simulink model "AB_Final_of_MPC_Bandwidth_Result_UnbalancedNew"  (R2022b)
settings: Solver=FixedStepDiscrete  StartTime=0.0  StopTime=Inf  FixedStep=100e-6  RelTol=1e-3  EnableMultiTasking=on
undefined symbols (not defined in the file): C28x, CPU1, CPU2, CurrentBypassValue, DiscIntNeverNeededParam, Down, GPTRIP1SEL, TZ1, Up
libraries: c2802xlib x20, simulink x17, dspstat3 x13, eeGeneralControl x10, c2837xDlib x5, c280xlib x5, PID_Lib x4, c2000lib x1, spsAlphaBetaZerotoabcLib x1
(part 8 of 10)

== system AB_Final_of_MPC_Bandwidth_Result_UnbalancedNew/Subsystem1/GridCurrentSecondPrediction/CostFunctionofVoltageVectors/CostFunctionVoltage4 ==
  MPCC_f32DGridCurrent_K_1 : Inport
  MPCC_f32QGridCurrent_K_1 : Inport  Port=2
  MPCC_f32DGridVoltage : Inport  Port=3
  MPCC_f32QGridVoltage : Inport  Port=4
  MPCC_f32Predictionterm_A : Inport  Port=5
  MPCC_f32Predictionterm_B : Inport  Port=6
  MPCC_f32Predictionterm_C : Inport  Port=7
  MPCC_f32DGridCurrentReference : Inport  Port=8
  MPCC_f32QGridCurrentReference : Inport  Port=9
  MPCC_f32DVoltageVector4 : Inport  Port=10
  MPCC_f32QVoltageVector4 : Inport  Port=11
  MPCC_f32DGridCurrent : Inport  Port=12
  MPCC_f32QGridCurrent : Inport  Port=13
  MPCC_f32DGridCurrent1 : Inport  Port=14
  MPCC_f32QGridCurrent1 : Inport  Port=15
  CostFunctionVoltage4 : Subsystem
  DGridCurrentSecondPrediction_Voltage4 : Subsystem
  QGridCurrentSecondPrediction_Voltage4 : Subsystem
  MPCC_f32CostFunction_Voltage4 : Outport
  wires:
  [MPCC_f32Predictionterm_B] -> QGridCurrentSecondPrediction_Voltage4/2(MPCC_f32Predictionterm_B)
  [MPCC_f32QGridCurrent_K_1] -> DGridCurrentSecondPrediction_Voltage4/5(MPCC_f32QGridCurrent_K_1)
  [MPCC_f32Predictionterm_A] -> QGridCurrentSecondPrediction_Voltage4/1(MPCC_f32Predictionterm_A)
  [MPCC_f32QGridCurrent_K_1] -> QGridCurrentSecondPrediction_Voltage4/5(MPCC_f32QGridCurrent_K_1)
  [MPCC_f32Predictionterm_B] -> DGridCurrentSecondPrediction_Voltage4/2(MPCC_f32Predictionterm_B)
  [MPCC_f32DGridCurrent_K_1] -> QGridCurrentSecondPrediction_Voltage4/4(MPCC_f32DGridCurrent_K_1)
  [MPCC_f32Predictionterm_C] -> QGridCurrentSecondPrediction_Voltage4/3(MPCC_f32Predictionterm_C)
  [MPCC_f32Predictionterm_A] -> DGridCurrentSecondPrediction_Voltage4/1(MPCC_f32Predictionterm_A)
  DGridCurrentSecondPrediction_Voltage4/1(MPCC_f32DGridCurrent_K_2_Voltage4) -> [MPCC_f32DGridCurrent_K_2_Voltage4]
  [MPCC_f32Predictionterm_C] -> DGridCurrentSecondPrediction_Voltage4/3(MPCC_f32Predictionterm_C)
  [MPCC_f32QGridVoltage] -> QGridCurrentSecondPrediction_Voltage4/6(MPCC_f32QGridVoltage)
  [MPCC_f32DGridVoltage] -> DGridCurrentSecondPrediction_Voltage4/6(MPCC_f32DGridVoltage)
  [MPCC_f32DGridCurrent_K_1] -> DGridCurrentSecondPrediction_Voltage4/4(MPCC_f32DGridCurrent_K_1)
  MPCC_f32QGridVoltage/1 -> [MPCC_f32QGridVoltage]
  MPCC_f32DGridCurrent_K_1/1 -> [MPCC_f32DGridCurrent_K_1]
  MPCC_f32Predictionterm_A/1 -> [MPCC_f32Predictionterm_A]
  MPCC_f32DGridVoltage/1 -> [MPCC_f32DGridVoltage]
  MPCC_f32Predictionterm_C/1 -> [MPCC_f32Predictionterm_C]
  MPCC_f32QGridCurrent_K_1/1 -> [MPCC_f32QGridCurrent_K_1]
  MPCC_f32Predictionterm_B/1 -> [MPCC_f32Predictionterm_B]
  MPCC_f32DGridCurrentReference/1 -> [MPCC_f32DGridCurrentReference]
  MPCC_f32QGridCurrentReference/1 -> [MPCC_f32QGridCurrentReference]
  QGridCurrentSecondPrediction_Voltage4/1(MPCC_f32QGridCurrent_K_2_Voltage4) -> [MPCC_f32QGridCurrent_K_2_Voltage4]
  CostFunctionVoltage4/1(MPCC_f32CostFunction_Voltage4) -> MPCC_f32CostFunction_Voltage4/1
  [MPCC_f32DGridCurrentReference] -> CostFunctionVoltage4/1(MPCC_f32DGridCurrentReference)
  [MPCC_f32QGridCurrentReference] -> CostFunctionVoltage4/2(MPCC_f32QGridCurrentReference)
  [MPCC_f32DGridCurrent_K_2_Voltage4] -> CostFunctionVoltage4/3(MPCC_f32DGridCurrent_K_2_Voltage4)
  [MPCC_f32QGridCurrent_K_2_Voltage4] -> CostFunctionVoltage4/4(MPCC_f32QGridCurrent_K_2_Voltage4)
  [MPCC_f32DGridCurrent] -> CostFunctionVoltage4/5(MPCC_f32DGridCurrent)
  [MPCC_f32QGridCurrent] -> CostFunctionVoltage4/6(MPCC_f32QGridCurrent)
  [MPCC_f32DVoltageVector4] -> DGridCurrentSecondPrediction_Voltage4/7(MPCC_f32DVoltageVector4)
  [MPCC_f32QVoltageVector4] -> QGridCurrentSecondPrediction_Voltage4/7(MPCC_f32QVoltageVector4)
  MPCC_f32DVoltageVector4/1 -> [MPCC_f32DVoltageVector4]
  MPCC_f32QVoltageVector4/1 -> [MPCC_f32QVoltageVector4]
  MPCC_f32QGridCurrent/1 -> [MPCC_f32QGridCurrent]
  MPCC_f32DGridCurrent/1 -> [MPCC_f32DGridCurrent]
  MPCC_f32DGridCurrent1/1 -> CostFunctionVoltage4/7(MPCC_f32DGridCurrent1)
  MPCC_f32QGridCurrent1/1 -> CostFunctionVoltage4/8(MPCC_f32QGridCurrent1)

== system AB_Final_of_MPC_Bandwidth_Result_UnbalancedNew/Subsystem1/GridCurrentSecondPrediction/CostFunctionofVoltageVectors/CostFunctionVoltage5 ==
  MPCC_f32DGridCurrent_K_1 : Inport
  MPCC_f32QGridCurrent_K_1 : Inport  Port=2
  MPCC_f32DGridVoltage : Inport  Port=3
  MPCC_f32QGridVoltage : Inport  Port=4
  MPCC_f32Predictionterm_A : Inport  Port=5
  MPCC_f32Predictionterm_B : Inport  Port=6
  MPCC_f32Predictionterm_C : Inport  Port=7
  MPCC_f32DGridCurrentReference : Inport  Port=8
  MPCC_f32QGridCurrentReference : Inport  Port=9
  MPCC_f32DVoltageVector5 : Inport  Port=10
  MPCC_f32QVoltageVector5 : Inport  Port=11
  MPCC_f32DGridCurrent : Inport  Port=12
  MPCC_f32QGridCurrent : Inport  Port=13
  MPCC_f32DGridCurrent1 : Inport  Port=14
  MPCC_f32QGridCurrent1 : Inport  Port=15
  CostFunctionVoltage5 : Subsystem
  DGridCurrentSecondPrediction_Voltage5 : Subsystem
  QGridCurrentSecondPrediction_Voltage5 : Subsystem
  MPCC_f32CostFunction_Voltage5 : Outport
  wires:
  [MPCC_f32Predictionterm_B] -> QGridCurrentSecondPrediction_Voltage5/2(MPCC_f32Predictionterm_B)
  [MPCC_f32QGridCurrent_K_1] -> DGridCurrentSecondPrediction_Voltage5/5(MPCC_f32QGridCurrent_K_1)
  [MPCC_f32Predictionterm_A] -> QGridCurrentSecondPrediction_Voltage5/1(MPCC_f32Predictionterm_A)
  [MPCC_f32QGridCurrent_K_1] -> QGridCurrentSecondPrediction_Voltage5/5(MPCC_f32QGridCurrent_K_1)
  [MPCC_f32Predictionterm_B] -> DGridCurrentSecondPrediction_Voltage5/2(MPCC_f32Predictionterm_B)
  [MPCC_f32DGridCurrent_K_1] -> QGridCurrentSecondPrediction_Voltage5/4(MPCC_f32DGridCurrent_K_1)
  [MPCC_f32Predictionterm_C] -> QGridCurrentSecondPrediction_Voltage5/3(MPCC_f32Predictionterm_C)
  [MPCC_f32Predictionterm_A] -> DGridCurrentSecondPrediction_Voltage5/1(MPCC_f32Predictionterm_A)
  DGridCurrentSecondPrediction_Voltage5/1(MPCC_f32DGridCurrent_K_2_Voltage5) -> [MPCC_f32DGridCurrent_K_2_Voltage5]
  [MPCC_f32Predictionterm_C] -> DGridCurrentSecondPrediction_Voltage5/3(MPCC_f32Predictionterm_C)
  [MPCC_f32QGridVoltage] -> QGridCurrentSecondPrediction_Voltage5/6(MPCC_f32QGridVoltage)
  [MPCC_f32DGridVoltage] -> DGridCurrentSecondPrediction_Voltage5/6(MPCC_f32DGridVoltage)
  [MPCC_f32DGridCurrent_K_1] -> DGridCurrentSecondPrediction_Voltage5/4(MPCC_f32DGridCurrent_K_1)
  MPCC_f32QGridVoltage/1 -> [MPCC_f32QGridVoltage]
  MPCC_f32DGridCurrent_K_1/1 -> [MPCC_f32DGridCurrent_K_1]
  MPCC_f32Predictionterm_A/1 -> [MPCC_f32Predictionterm_A]
  MPCC_f32DGridVoltage/1 -> [MPCC_f32DGridVoltage]
  MPCC_f32Predictionterm_C/1 -> [MPCC_f32Predictionterm_C]
  MPCC_f32QGridCurrent_K_1/1 -> [MPCC_f32QGridCurrent_K_1]
  MPCC_f32Predictionterm_B/1 -> [MPCC_f32Predictionterm_B]
  MPCC_f32DGridCurrentReference/1 -> [MPCC_f32DGridCurrentReference]
  MPCC_f32QGridCurrentReference/1 -> [MPCC_f32QGridCurrentReference]
  QGridCurrentSecondPrediction_Voltage5/1(MPCC_f32QGridCurrent_K_2_Voltage5) -> [MPCC_f32QGridCurrent_K_2_Voltage5]
  CostFunctionVoltage5/1(MPCC_f32CostFunction_Voltage5) -> MPCC_f32CostFunction_Voltage5/1
  [MPCC_f32DGridCurrentReference] -> CostFunctionVoltage5/1(MPCC_f32DGridCurrentReference)
  [MPCC_f32QGridCurrentReference] -> CostFunctionVoltage5/2(MPCC_f32QGridCurrentReference)
  [MPCC_f32DGridCurrent_K_2_Voltage5] -> CostFunctionVoltage5/3(MPCC_f32DGridCurrent_K_2_Voltage5)
  [MPCC_f32QGridCurrent_K_2_Voltage5] -> CostFunctionVoltage5/4(MPCC_f32QGridCurrent_K_2_Voltage5)
  [MPCC_f32DGridCurrent] -> CostFunctionVoltage5/5(MPCC_f32DGridCurrent)
  [MPCC_f32QGridCurrent] -> CostFunctionVoltage5/6(MPCC_f32QGridCurrent)
  [MPCC_f32DVoltageVector5] -> DGridCurrentSecondPrediction_Voltage5/7(MPCC_f32DVoltageVector5)
  [MPCC_f32QVoltageVector5] -> QGridCurrentSecondPrediction_Voltage5/7(MPCC_f32QVoltageVector5)
  MPCC_f32DVoltageVector5/1 -> [MPCC_f32DVoltageVector5]
  MPCC_f32QVoltageVector5/1 -> [MPCC_f32QVoltageVector5]
  MPCC_f32QGridCurrent/1 -> [MPCC_f32QGridCurrent]
  MPCC_f32DGridCurrent/1 -> [MPCC_f32DGridCurrent]
  MPCC_f32DGridCurrent1/1 -> CostFunctionVoltage5/7(MPCC_f32DGridCurrent1)
  MPCC_f32QGridCurrent1/1 -> CostFunctionVoltage5/8(MPCC_f32QGridCurrent1)

== system AB_Final_of_MPC_Bandwidth_Result_UnbalancedNew/Subsystem1/GridCurrentSecondPrediction/CostFunctionofVoltageVectors/CostFunctionVoltage6 ==
  MPCC_f32DGridCurrent_K_1 : Inport
  MPCC_f32QGridCurrent_K_1 : Inport  Port=2
  MPCC_f32DGridVoltage : Inport  Port=3
  MPCC_f32QGridVoltage : Inport  Port=4
  MPCC_f32Predictionterm_A : Inport  Port=5
  MPCC_f32Predictionterm_B : Inport  Port=6
  MPCC_f32Predictionterm_C : Inport  Port=7
  MPCC_f32DGridCurrentReference : Inport  Port=8
  MPCC_f32QGridCurrentReference : Inport  Port=9
  MPCC_f32DVoltageVector6 : Inport  Port=10
  MPCC_f32QVoltageVector6 : Inport  Port=11
  MPCC_f32DGridCurrent : Inport  Port=12
  MPCC_f32QGridCurrent : Inport  Port=13
  MPCC_f32DGridCurrent1 : Inport  Port=14
  MPCC_f32QGridCurrent1 : Inport  Port=15
  CostFunctionVoltage6 : Subsystem
  DGridCurrentSecondPrediction_Voltage6 : Subsystem
  QGridCurrentSecondPrediction_Voltage6 : Subsystem
  MPCC_f32CostFunction_Voltage6 : Outport
  wires:
  [MPCC_f32Predictionterm_B] -> QGridCurrentSecondPrediction_Voltage6/2(MPCC_f32Predictionterm_B)
  [MPCC_f32QGridCurrent_K_1] -> DGridCurrentSecondPrediction_Voltage6/5(MPCC_f32QGridCurrent_K_1)
  [MPCC_f32Predictionterm_A] -> QGridCurrentSecondPrediction_Voltage6/1(MPCC_f32Predictionterm_A)
  [MPCC_f32QGridCurrent_K_1] -> QGridCurrentSecondPrediction_Voltage6/5(MPCC_f32QGridCurrent_K_1)
  [MPCC_f32Predictionterm_B] -> DGridCurrentSecondPrediction_Voltage6/2(MPCC_f32Predictionterm_B)
  [MPCC_f32DGridCurrent_K_1] -> QGridCurrentSecondPrediction_Voltage6/4(MPCC_f32DGridCurrent_K_1)
  [MPCC_f32Predictionterm_C] -> QGridCurrentSecondPrediction_Voltage6/3(MPCC_f32Predictionterm_C)
  [MPCC_f32Predictionterm_A] -> DGridCurrentSecondPrediction_Voltage6/1(MPCC_f32Predictionterm_A)
  DGridCurrentSecondPrediction_Voltage6/1(MPCC_f32DGridCurrent_K_2_Voltage6) -> [MPCC_f32DGridCurrent_K_2_Voltage6]
  [MPCC_f32Predictionterm_C] -> DGridCurrentSecondPrediction_Voltage6/3(MPCC_f32Predictionterm_C)
  [MPCC_f32QGridVoltage] -> QGridCurrentSecondPrediction_Voltage6/6(MPCC_f32QGridVoltage)
  [MPCC_f32DGridVoltage] -> DGridCurrentSecondPrediction_Voltage6/6(MPCC_f32DGridVoltage)
  [MPCC_f32DGridCurrent_K_1] -> DGridCurrentSecondPrediction_Voltage6/4(MPCC_f32DGridCurrent_K_1)
  MPCC_f32QGridVoltage/1 -> [MPCC_f32QGridVoltage]
  MPCC_f32DGridCurrent_K_1/1 -> [MPCC_f32DGridCurrent_K_1]
  MPCC_f32Predictionterm_A/1 -> [MPCC_f32Predictionterm_A]
  MPCC_f32DGridVoltage/1 -> [MPCC_f32DGridVoltage]
  MPCC_f32Predictionterm_C/1 -> [MPCC_f32Predictionterm_C]
  MPCC_f32QGridCurrent_K_1/1 -> [MPCC_f32QGridCurrent_K_1]
  MPCC_f32Predictionterm_B/1 -> [MPCC_f32Predictionterm_B]
  MPCC_f32DGridCurrentReference/1 -> [MPCC_f32DGridCurrentReference]
  MPCC_f32QGridCurrentReference/1 -> [MPCC_f32QGridCurrentReference]
  QGridCurrentSecondPrediction_Voltage6/1(MPCC_f32QGridCurrent_K_2_Voltage6) -> [MPCC_f32QGridCurrent_K_2_Voltage6]
  CostFunctionVoltage6/1(MPCC_f32CostFunction_Voltage6) -> MPCC_f32CostFunction_Voltage6/1
  [MPCC_f32DGridCurrentReference] -> CostFunctionVoltage6/1(MPCC_f32DGridCurrentReference)
  [MPCC_f32QGridCurrentReference] -> CostFunctionVoltage6/2(MPCC_f32QGridCurrentReference)
  [MPCC_f32DGridCurrent_K_2_Voltage6] -> CostFunctionVoltage6/3(MPCC_f32DGridCurrent_K_2_Voltage6)
  [MPCC_f32QGridCurrent_K_2_Voltage6] -> CostFunctionVoltage6/4(MPCC_f32QGridCurrent_K_2_Voltage6)
  [MPCC_f32DGridCurrent] -> CostFunctionVoltage6/5(MPCC_f32DGridCurrent)
  [MPCC_f32QGridCurrent] -> CostFunctionVoltage6/6(MPCC_f32QGridCurrent)
  [MPCC_f32DVoltageVector6] -> DGridCurrentSecondPrediction_Voltage6/7(MPCC_f32DVoltageVector6)
  [MPCC_f32QVoltageVector6] -> QGridCurrentSecondPrediction_Voltage6/7(MPCC_f32QVoltageVector6)
  MPCC_f32DVoltageVector6/1 -> [MPCC_f32DVoltageVector6]
  MPCC_f32QVoltageVector6/1 -> [MPCC_f32QVoltageVector6]
  MPCC_f32QGridCurrent/1 -> [MPCC_f32QGridCurrent]
  MPCC_f32DGridCurrent/1 -> [MPCC_f32DGridCurrent]
  MPCC_f32DGridCurrent1/1 -> CostFunctionVoltage6/7(MPCC_f32DGridCurrent1)
  MPCC_f32QGridCurrent1/1 -> CostFunctionVoltage6/8(MPCC_f32QGridCurrent1)

== system AB_Final_of_MPC_Bandwidth_Result_UnbalancedNew/Subsystem1/GridCurrentSecondPrediction/CostFunctionofVoltageVectors/DQVoltageVector1 ==
  MPCC_f32ElectricalAngle_K_1 : Inport
  MPCC_f32AlphaConvVoltage1 : Inport  Port=2
  MPCC_f32BetaConvVoltage1 : Inport  Port=3
  Add : Sum
  Add1 : Sum  Inputs=+-
  Product{,1..3} (4 alike) : Product
  Sin : Trigonometry  Operator=cos
  Sin1 : Trigonometry
  Sin2 : Trigonometry  Operator=cos
  Sin3 : Trigonometry
  MPCC_f32DVoltageVector1 : Outport
  MPCC_f32QVoltageVector1 : Outport  Port=2
  wires:
  Sin2/1 -> Product2/1
  [MPCC_f32AlphaConvVoltage1] -> Product3/2
  Sin1/1 -> Product1/1
  Sin3/1 -> Product3/1
  Product/1 -> Add/1
  [MPCC_f32BetaConvVoltage1] -> Product2/2
  [MPCC_f32ElectricalAngle_K_1] -> Sin2/1
  [MPCC_f32BetaConvVoltage1] -> Product1/2
  Product2/1 -> Add1/1
  Product3/1 -> Add1/2
  [MPCC_f32ElectricalAngle_K_1] -> Sin3/1
  MPCC_f32ElectricalAngle_K_1/1 -> [MPCC_f32ElectricalAngle_K_1]
  [MPCC_f32ElectricalAngle_K_1] -> Sin/1
  [MPCC_f32AlphaConvVoltage1] -> Product/2
  Product1/1 -> Add/2
  Sin/1 -> Product/1
  [MPCC_f32ElectricalAngle_K_1] -> Sin1/1
  MPCC_f32AlphaConvVoltage1/1 -> MPCC_f32DVoltageVector1/1, [MPCC_f32AlphaConvVoltage1]
  MPCC_f32BetaConvVoltage1/1 -> MPCC_f32QVoltageVector1/1, [MPCC_f32BetaConvVoltage1]

== system AB_Final_of_MPC_Bandwidth_Result_UnbalancedNew/Subsystem1/GridCurrentSecondPrediction/CostFunctionofVoltageVectors/DQVoltageVector2 ==
  MPCC_f32ElectricalAngle_K_1 : Inport
  MPCC_f32AlphaConvVoltage2 : Inport  Port=2
  MPCC_f32BetaConvVoltage2 : Inport  Port=3
  Add : Sum
  Add1 : Sum  Inputs=+-
  Product{,1..3} (4 alike) : Product
  Sin : Trigonometry  Operator=cos
  Sin1 : Trigonometry
  Sin2 : Trigonometry  Operator=cos
  Sin3 : Trigonometry
  MPCC_f32DVoltageVector2 : Outport
  MPCC_f32QVoltageVector2 : Outport  Port=2
  wires:
  Sin2/1 -> Product2/1
  [MPCC_f32AlphaConvVoltage2] -> Product3/2
  Sin1/1 -> Product1/1
  Sin3/1 -> Product3/1
  Product/1 -> Add/1
  [MPCC_f32BetaConvVoltage2] -> Product2/2
  [MPCC_f32ElectricalAngle_K_1] -> Sin2/1
  [MPCC_f32BetaConvVoltage2] -> Product1/2
  Product2/1 -> Add1/1
  Product3/1 -> Add1/2
  [MPCC_f32ElectricalAngle_K_1] -> Sin3/1
  MPCC_f32ElectricalAngle_K_1/1 -> [MPCC_f32ElectricalAngle_K_1]
  [MPCC_f32ElectricalAngle_K_1] -> Sin/1
  [MPCC_f32AlphaConvVoltage2] -> Product/2
  Product1/1 -> Add/2
  Sin/1 -> Product/1
  [MPCC_f32ElectricalAngle_K_1] -> Sin1/1
  MPCC_f32AlphaConvVoltage2/1 -> MPCC_f32DVoltageVector2/1, [MPCC_f32AlphaConvVoltage2]
  MPCC_f32BetaConvVoltage2/1 -> MPCC_f32QVoltageVector2/1, [MPCC_f32BetaConvVoltage2]

== system AB_Final_of_MPC_Bandwidth_Result_UnbalancedNew/Subsystem1/GridCurrentSecondPrediction/CostFunctionofVoltageVectors/DQVoltageVector3 ==
  MPCC_f32ElectricalAngle_K_1 : Inport
  MPCC_f32AlphaConvVoltage3 : Inport  Port=2
  MPCC_f32BetaConvVoltage3 : Inport  Port=3
  Add : Sum
  Add1 : Sum  Inputs=+-
  Product{,1..3} (4 alike) : Product
  Sin : Trigonometry  Operator=cos
  Sin1 : Trigonometry
  Sin2 : Trigonometry  Operator=cos
  Sin3 : Trigonometry
  MPCC_f32DVoltageVector3 : Outport
  MPCC_f32QVoltageVector3 : Outport  Port=2
  wires:
  Sin2/1 -> Product2/1
  [MPCC_f32AlphaConvVoltage3] -> Product3/2
  Sin1/1 -> Product1/1
  Sin3/1 -> Product3/1
  Product/1 -> Add/1
  [MPCC_f32BetaConvVoltage3] -> Product2/2
  [MPCC_f32ElectricalAngle_K_1] -> Sin2/1
  [MPCC_f32BetaConvVoltage3] -> Product1/2
  Product2/1 -> Add1/1
  Product3/1 -> Add1/2
  [MPCC_f32ElectricalAngle_K_1] -> Sin3/1
  MPCC_f32ElectricalAngle_K_1/1 -> [MPCC_f32ElectricalAngle_K_1]
  [MPCC_f32ElectricalAngle_K_1] -> Sin/1
  [MPCC_f32AlphaConvVoltage3] -> Product/2
  Product1/1 -> Add/2
  Sin/1 -> Product/1
  [MPCC_f32ElectricalAngle_K_1] -> Sin1/1
  MPCC_f32AlphaConvVoltage3/1 -> MPCC_f32DVoltageVector3/1, [MPCC_f32AlphaConvVoltage3]
  MPCC_f32BetaConvVoltage3/1 -> MPCC_f32QVoltageVector3/1, [MPCC_f32BetaConvVoltage3]

== system AB_Final_of_MPC_Bandwidth_Result_UnbalancedNew/Subsystem1/GridCurrentSecondPrediction/CostFunctionofVoltageVectors/DQVoltageVector4 ==
  MPCC_f32ElectricalAngle_K_1 : Inport
  MPCC_f32AlphaConvVoltage4 : Inport  Port=2
  MPCC_f32BetaConvVoltage4 : Inport  Port=3
  Add : Sum
  Add1 : Sum  Inputs=+-
  Product{,1..3} (4 alike) : Product
  Sin : Trigonometry  Operator=cos
  Sin1 : Trigonometry
  Sin2 : Trigonometry  Operator=cos
  Sin3 : Trigonometry
  MPCC_f32DVoltageVector4 : Outport
  MPCC_f32QVoltageVector4 : Outport  Port=2
  wires:
  Sin2/1 -> Product2/1
  [MPCC_f32AlphaConvVoltage4] -> Product3/2
  Sin1/1 -> Product1/1
  Sin3/1 -> Product3/1
  Product/1 -> Add/1
  [MPCC_f32BetaConvVoltage4] -> Product2/2
  [MPCC_f32ElectricalAngle_K_1] -> Sin2/1
  [MPCC_f32BetaConvVoltage4] -> Product1/2
  Product2/1 -> Add1/1
  Product3/1 -> Add1/2
  [MPCC_f32ElectricalAngle_K_1] -> Sin3/1
  MPCC_f32ElectricalAngle_K_1/1 -> [MPCC_f32ElectricalAngle_K_1]
  [MPCC_f32ElectricalAngle_K_1] -> Sin/1
  [MPCC_f32AlphaConvVoltage4] -> Product/2
  Product1/1 -> Add/2
  Sin/1 -> Product/1
  [MPCC_f32ElectricalAngle_K_1] -> Sin1/1
  MPCC_f32AlphaConvVoltage4/1 -> MPCC_f32DVoltageVector4/1, [MPCC_f32AlphaConvVoltage4]
  MPCC_f32BetaConvVoltage4/1 -> MPCC_f32QVoltageVector4/1, [MPCC_f32BetaConvVoltage4]

== system AB_Final_of_MPC_Bandwidth_Result_UnbalancedNew/Subsystem1/GridCurrentSecondPrediction/CostFunctionofVoltageVectors/DQVoltageVector5 ==
  MPCC_f32ElectricalAngle_K_1 : Inport
  MPCC_f32AlphaConvVoltage5 : Inport  Port=2
  MPCC_f32BetaConvVoltage5 : Inport  Port=3
  Add : Sum
  Add1 : Sum  Inputs=+-
  Product{,1..3} (4 alike) : Product
  Sin : Trigonometry  Operator=cos
  Sin1 : Trigonometry
  Sin2 : Trigonometry  Operator=cos
  Sin3 : Trigonometry
  MPCC_f32DVoltageVector5 : Outport
  MPCC_f32QVoltageVector5 : Outport  Port=2
  wires:
  Sin2/1 -> Product2/1
  [MPCC_f32AlphaConvVoltage5] -> Product3/2
  Sin1/1 -> Product1/1
  Sin3/1 -> Product3/1
  Product/1 -> Add/1
  [MPCC_f32BetaConvVoltage5] -> Product2/2
  [MPCC_f32ElectricalAngle_K_1] -> Sin2/1
  [MPCC_f32BetaConvVoltage5] -> Product1/2
  Product2/1 -> Add1/1
  Product3/1 -> Add1/2
  [MPCC_f32ElectricalAngle_K_1] -> Sin3/1
  MPCC_f32ElectricalAngle_K_1/1 -> [MPCC_f32ElectricalAngle_K_1]
  [MPCC_f32ElectricalAngle_K_1] -> Sin/1
  [MPCC_f32AlphaConvVoltage5] -> Product/2
  Product1/1 -> Add/2
  Sin/1 -> Product/1
  [MPCC_f32ElectricalAngle_K_1] -> Sin1/1
  MPCC_f32AlphaConvVoltage5/1 -> MPCC_f32DVoltageVector5/1, [MPCC_f32AlphaConvVoltage5]
  MPCC_f32BetaConvVoltage5/1 -> MPCC_f32QVoltageVector5/1, [MPCC_f32BetaConvVoltage5]

== system AB_Final_of_MPC_Bandwidth_Result_UnbalancedNew/Subsystem1/GridCurrentSecondPrediction/CostFunctionofVoltageVectors/DQVoltageVector6 ==
  MPCC_f32ElectricalAngle_K_1 : Inport
  MPCC_f32AlphaConvVoltage6 : Inport  Port=2
  MPCC_f32BetaConvVoltage6 : Inport  Port=3
  Add : Sum
  Add1 : Sum  Inputs=+-
  Product{,1..3} (4 alike) : Product
  Sin : Trigonometry  Operator=cos
  Sin1 : Trigonometry
  Sin2 : Trigonometry  Operator=cos
  Sin3 : Trigonometry
  MPCC_f32DVoltageVector6 : Outport
  MPCC_f32QVoltageVector6 : Outport  Port=2
  wires:
  Sin2/1 -> Product2/1
  [MPCC_f32AlphaConvVoltage6] -> Product3/2
  Sin1/1 -> Product1/1
  Sin3/1 -> Product3/1
  Product/1 -> Add/1
  [MPCC_f32BetaConvVoltage6] -> Product2/2
  [MPCC_f32ElectricalAngle_K_1] -> Sin2/1
  [MPCC_f32BetaConvVoltage6] -> Product1/2
  Product2/1 -> Add1/1
  Product3/1 -> Add1/2
  [MPCC_f32ElectricalAngle_K_1] -> Sin3/1
  MPCC_f32ElectricalAngle_K_1/1 -> [MPCC_f32ElectricalAngle_K_1]
  [MPCC_f32ElectricalAngle_K_1] -> Sin/1
  [MPCC_f32AlphaConvVoltage6] -> Product/2
  Product1/1 -> Add/2
  Sin/1 -> Product/1
  [MPCC_f32ElectricalAngle_K_1] -> Sin1/1
  MPCC_f32AlphaConvVoltage6/1 -> MPCC_f32DVoltageVector6/1, [MPCC_f32AlphaConvVoltage6]
  MPCC_f32BetaConvVoltage6/1 -> MPCC_f32QVoltageVector6/1, [MPCC_f32BetaConvVoltage6]

== system AB_Final_of_MPC_Bandwidth_Result_UnbalancedNew/Subsystem1/ModulatorTimes/ConverterVoltage/DQConvSector1 ==
  MPCC_f32ElectricalAngle_K_1 : Inport
  MPCC_f32AlphaConvVoltage1 : Inport  Port=2
  MPCC_f32BetaConvVoltage1 : Inport  Port=3
  MPCC_f32AlphaConvVoltage2 : Inport  Port=4
  MPCC_f32BetaConvVoltage2 : Inport  Port=5
  MPCC_f32Duty_Sector1 : Inport  Port=6
  Add : Sum  Commented=on
  Add1 : Sum  Commented=on  Inputs=-+
  Add2 : Sum
  Add3 : Sum
  Demux : Demux
  From1 : From  Commented=on  GotoTag=MPCC_f32AlphaConvSector1
  From2 : From  Commented=on  GotoTag=MPCC_f32BetaConvSector1
  From{3,6..8} (4 alike) : From  Commented=on  GotoTag=MPCC_f32ElectricalAngle_K_1
  From4 : From  Commented=on  GotoTag=MPCC_f32AlphaConvSector1
  From5 : From  Commented=on  GotoTag=MPCC_f32BetaConvSector1
  Product{,1..3} (4 alike) : Product  Commented=on
  Product{4..7} (4 alike) : Product
  Sin : Trigonometry  Commented=on  Operator=cos
  Sin1 : Trigonometry  Commented=on
  Sin2 : Trigonometry  Commented=on
  Sin3 : Trigonometry  Commented=on  Operator=cos
  MPCC_f32DConvSector1 : Outport
  MPCC_f32QConvSector1 : Outport  Port=2
  wires:
  Sin2/1 -> Product2/1
  From5/1 -> Product3/2
  Sin1/1 -> Product1/1
  Sin3/1 -> Product3/1
  Product/1 -> Add/1
  From4/1 -> Product2/2
  From8/1 -> Sin2/1
  From2/1 -> Product1/2
  Add1/1 -> ?
  Product2/1 -> Add1/1
  Product3/1 -> Add1/2
  From6/1 -> Sin3/1
  MPCC_f32ElectricalAngle_K_1/1 -> [MPCC_f32ElectricalAngle_K_1]
  Add/1 -> ?
  From7/1 -> Sin/1
  From1/1 -> Product/2
  Product1/1 -> Add/2
  Sin/1 -> Product/1
  From3/1 -> Sin1/1
  MPCC_f32AlphaConvVoltage1/1 -> [MPCC_f32AlphaConvVoltage1]
  MPCC_f32BetaConvVoltage1/1 -> [MPCC_f32BetaConvVoltage1]
  MPCC_f32AlphaConvVoltage2/1 -> [MPCC_f32AlphaConvVoltage2]
  MPCC_f32BetaConvVoltage2/1 -> [MPCC_f32BetaConvVoltage2]
  Add2/1 -> MPCC_f32DConvSector1/1, [MPCC_f32AlphaConvSector1]
  [MPCC_f32DutyA_Sector1] -> Product4/1
  [MPCC_f32DutyB_Sector1] -> Product5/1
  [MPCC_f32AlphaConvVoltage1] -> Product4/2
  Product4/1 -> Add2/1
  [MPCC_f32AlphaConvVoltage2] -> Product5/2
  Product5/1 -> Add2/2
  [MPCC_f32DutyB_Sector1] -> Product7/1
  [MPCC_f32DutyA_Sector1] -> Product6/1
  [MPCC_f32BetaConvVoltage2] -> Product7/2
  Product6/1 -> Add3/1
  Product7/1 -> Add3/2
  [MPCC_f32BetaConvVoltage1] -> Product6/2
  Add3/1 -> MPCC_f32QConvSector1/1, [MPCC_f32BetaConvSector1]
  MPCC_f32Duty_Sector1/1 -> Demux/1
  Demux/1 -> [MPCC_f32DutyA_Sector1]
  Demux/2 -> [MPCC_f32DutyB_Sector1]

== system AB_Final_of_MPC_Bandwidth_Result_UnbalancedNew/Subsystem1/ModulatorTimes/ConverterVoltage/DQConvSector2 ==
  MPCC_f32ElectricalAngle_K_1 : Inport
  MPCC_f32AlphaConvVoltage2 : Inport  Port=2
  MPCC_f32BetaConvVoltage2 : Inport  Port=3
  MPCC_f32AlphaConvVoltage3 : Inport  Port=4
  MPCC_f32BetaConvVoltage3 : Inport  Port=5
  MPCC_f32Duty_Sector2 : Inport  Port=6
  Add : Sum  Commented=on
  Add1 : Sum  Commented=on  Inputs=-+
  Add2 : Sum
  Add3 : Sum
  Demux : Demux
  From1 : From  Commented=on  GotoTag=MPCC_f32AlphaConvSector2
  From2 : From  Commented=on  GotoTag=MPCC_f32BetaConvSector2
  From{3,6..8} (4 alike) : From  Commented=on  GotoTag=MPCC_f32ElectricalAngle_K_1
  From4 : From  Commented=on  GotoTag=MPCC_f32AlphaConvSector2
  From5 : From  Commented=on  GotoTag=MPCC_f32BetaConvSector2
  Product{,1..3} (4 alike) : Product  Commented=on
  Product{4..7} (4 alike) : Product
  Sin : Trigonometry  Commented=on  Operator=cos
  Sin1 : Trigonometry  Commented=on
  Sin2 : Trigonometry  Commented=on
  Sin3 : Trigonometry  Commented=on  Operator=cos
  MPCC_f32DConvSector2 : Outport
  MPCC_f32QConvSector2 : Outport  Port=2
  wires:
  Sin2/1 -> Product2/1
  From5/1 -> Product3/2
  Sin1/1 -> Product1/1
  Sin3/1 -> Product3/1
  Product/1 -> Add/1
  From4/1 -> Product2/2
  From8/1 -> Sin2/1
  From2/1 -> Product1/2
  Product2/1 -> Add1/1
  Product3/1 -> Add1/2
  From6/1 -> Sin3/1
  MPCC_f32ElectricalAngle_K_1/1 -> [MPCC_f32ElectricalAngle_K_1]
  From7/1 -> Sin/1
  From1/1 -> Product/2
  Product1/1 -> Add/2
  Sin/1 -> Product/1
  From3/1 -> Sin1/1
  MPCC_f32AlphaConvVoltage2/1 -> [MPCC_f32AlphaConvVoltage2]
  MPCC_f32BetaConvVoltage2/1 -> [MPCC_f32BetaConvVoltage2]
  MPCC_f32AlphaConvVoltage3/1 -> [MPCC_f32AlphaConvVoltage3]
  MPCC_f32BetaConvVoltage3/1 -> [MPCC_f32BetaConvVoltage3]
  [MPCC_f32DutyA_Sector2] -> Product4/1
  [MPCC_f32DutyB_Sector2] -> Product5/1
  [MPCC_f32AlphaConvVoltage2] -> Product4/2
  Product4/1 -> Add2/1
  [MPCC_f32AlphaConvVoltage3] -> Product5/2
  Product5/1 -> Add2/2
  [MPCC_f32DutyB_Sector2] -> Product7/1
  [MPCC_f32DutyA_Sector2] -> Product6/1
  [MPCC_f32BetaConvVoltage3] -> Product7/2
  Product6/1 -> Add3/1
  Product7/1 -> Add3/2
  [MPCC_f32BetaConvVoltage2] -> Product6/2
  MPCC_f32Duty_Sector2/1 -> Demux/1
  Demux/1 -> [MPCC_f32DutyA_Sector2]
  Demux/2 -> [MPCC_f32DutyB_Sector2]
  Add3/1 -> MPCC_f32QConvSector2/1, [MPCC_f32BetaConvSector2]
  Add2/1 -> MPCC_f32DConvSector2/1, [MPCC_f32AlphaConvSector2]

== system AB_Final_of_MPC_Bandwidth_Result_UnbalancedNew/Subsystem1/ModulatorTimes/ConverterVoltage/DQConvSector3 ==
  MPCC_f32ElectricalAngle_K_1 : Inport
  MPCC_f32AlphaConvVoltage3 : Inport  Port=2
  MPCC_f32BetaConvVoltage3 : Inport  Port=3
  MPCC_f32AlphaConvVoltage4 : Inport  Port=4
  MPCC_f32BetaConvVoltage4 : Inport  Port=5
  MPCC_f32Duty_Sector3 : Inport  Port=6
  Add : Sum  Commented=on
  Add1 : Sum  Commented=on  Inputs=-+
  Add2 : Sum
  Add3 : Sum
  Demux : Demux
  From1 : From  Commented=on  GotoTag=MPCC_f32AlphaConvSector3
  From2 : From  Commented=on  GotoTag=MPCC_f32BetaConvSector3
  From{3,6..8} (4 alike) : From  Commented=on  GotoTag=MPCC_f32ElectricalAngle_K_1
  From4 : From  Commented=on  GotoTag=MPCC_f32AlphaConvSector3
  From5 : From  Commented=on  GotoTag=MPCC_f32BetaConvSector3
  Product{,1..3} (4 alike) : Product  Commented=on
  Product{4..7} (4 alike) : Product
  Sin : Trigonometry  Commented=on  Operator=cos
  Sin1 : Trigonometry  Commented=on
  Sin2 : Trigonometry  Commented=on
  Sin3 : Trigonometry  Commented=on  Operator=cos
  MPCC_f32DConvSector3 : Outport
  MPCC_f32QConvSector3 : Outport  Port=2
  wires:
  Sin2/1 -> Product2/1
  From5/1 -> Product3/2
  Sin1/1 -> Product1/1
  Sin3/1 -> Product3/1
  Product/1 -> Add/1
  From4/1 -> Product2/2
  From8/1 -> Sin2/1
  From2/1 -> Product1/2
  Product2/1 -> Add1/1
  Product3/1 -> Add1/2
  From6/1 -> Sin3/1
  MPCC_f32ElectricalAngle_K_1/1 -> [MPCC_f32ElectricalAngle_K_1]
  From7/1 -> Sin/1
  From1/1 -> Product/2
  Product1/1 -> Add/2
  Sin/1 -> Product/1
  From3/1 -> Sin1/1
  MPCC_f32AlphaConvVoltage3/1 -> [MPCC_f32AlphaConvVoltage3]
  MPCC_f32BetaConvVoltage3/1 -> [MPCC_f32BetaConvVoltage3]
  MPCC_f32AlphaConvVoltage4/1 -> [MPCC_f32AlphaConvVoltage4]
  MPCC_f32BetaConvVoltage4/1 -> [MPCC_f32BetaConvVoltage4]
  [MPCC_f32DutyA_Sector3] -> Product4/1
  [MPCC_f32DutyB_Sector3] -> Product5/1
  [MPCC_f32AlphaConvVoltage3] -> Product4/2
  Product4/1 -> Add2/1
  [MPCC_f32AlphaConvVoltage4] -> Product5/2
  Product5/1 -> Add2/2
  [MPCC_f32DutyB_Sector3] -> Product7/1
  [MPCC_f32DutyA_Sector3] -> Product6/1
  [MPCC_f32BetaConvVoltage4] -> Product7/2
  Product6/1 -> Add3/1
  Product7/1 -> Add3/2
  [MPCC_f32BetaConvVoltage3] -> Product6/2
  MPCC_f32Duty_Sector3/1 -> Demux/1
  Demux/1 -> [MPCC_f32DutyA_Sector3]
  Demux/2 -> [MPCC_f32DutyB_Sector3]
  Add2/1 -> MPCC_f32DConvSector3/1, [MPCC_f32AlphaConvSector3]
  Add3/1 -> MPCC_f32QConvSector3/1, [MPCC_f32BetaConvSector3]

== system AB_Final_of_MPC_Bandwidth_Result_UnbalancedNew/Subsystem1/ModulatorTimes/ConverterVoltage/DQConvSector4 ==
  MPCC_f32ElectricalAngle_K_1 : Inport
  MPCC_f32AlphaConvVoltage4 : Inport  Port=2
  MPCC_f32BetaConvVoltage4 : Inport  Port=3
  MPCC_f32AlphaConvVoltage5 : Inport  Port=4
  MPCC_f32BetaConvVoltage5 : Inport  Port=5
  MPCC_f32Duty_Sector4 : Inport  Port=6
  Add : Sum  Commented=on
  Add1 : Sum  Commented=on  Inputs=-+
  Add2 : Sum
  Add3 : Sum
  Demux : Demux
  From1 : From  Commented=on  GotoTag=MPCC_f32AlphaConvSector4
  From2 : From  Commented=on  GotoTag=MPCC_f32BetaConvSector4
  From{3,6..8} (4 alike) : From  Commented=on  GotoTag=MPCC_f32ElectricalAngle_K_1
  From4 : From  Commented=on  GotoTag=MPCC_f32AlphaConvSector4
  From5 : From  Commented=on  GotoTag=MPCC_f32BetaConvSector4
  Product{,1..3} (4 alike) : Product  Commented=on
  Product{4..7} (4 alike) : Product
  Sin : Trigonometry  Commented=on  Operator=cos
  Sin1 : Trigonometry  Commented=on
  Sin2 : Trigonometry  Commented=on
  Sin3 : Trigonometry  Commented=on  Operator=cos
  MPCC_f32DConvSector4 : Outport
  MPCC_f32QConvSector4 : Outport  Port=2
  wires:
  Sin2/1 -> Product2/1
  From5/1 -> Product3/2
  Sin1/1 -> Product1/1
  Sin3/1 -> Product3/1
  Product/1 -> Add/1
  From4/1 -> Product2/2
  From8/1 -> Sin2/1
  From2/1 -> Product1/2
  Product2/1 -> Add1/1
  Product3/1 -> Add1/2
  From6/1 -> Sin3/1
  MPCC_f32ElectricalAngle_K_1/1 -> [MPCC_f32ElectricalAngle_K_1]
  From7/1 -> Sin/1
  From1/1 -> Product/2
  Product1/1 -> Add/2
  Sin/1 -> Product/1
  From3/1 -> Sin1/1
  MPCC_f32AlphaConvVoltage4/1 -> [MPCC_f32AlphaConvVoltage4]
  MPCC_f32BetaConvVoltage4/1 -> [MPCC_f32BetaConvVoltage4]
  MPCC_f32AlphaConvVoltage5/1 -> [MPCC_f32AlphaConvVoltage5]
  MPCC_f32BetaConvVoltage5/1 -> [MPCC_f32BetaConvVoltage5]
  [MPCC_f32DutyA_Sector4] -> Product4/1
  [MPCC_f32DutyB_Sector4] -> Product5/1
  [MPCC_f32AlphaConvVoltage4] -> Product4/2
  Product4/1 -> Add2/1
  [MPCC_f32AlphaConvVoltage5] -> Product5/2
  Product5/1 -> Add2/2
  [MPCC_f32DutyB_Sector4] -> Product7/1
  [MPCC_f32DutyA_Sector4] -> Product6/1
  [MPCC_f32BetaConvVoltage5] -> Product7/2
  Product6/1 -> Add3/1
  Product7/1 -> Add3/2
  [MPCC_f32BetaConvVoltage4] -> Product6/2
  MPCC_f32Duty_Sector4/1 -> Demux/1
  Demux/1 -> [MPCC_f32DutyA_Sector4]
  Demux/2 -> [MPCC_f32DutyB_Sector4]
  Add3/1 -> MPCC_f32QConvSector4/1, [MPCC_f32BetaConvSector4]
  Add2/1 -> MPCC_f32DConvSector4/1, [MPCC_f32AlphaConvSector4]

== system AB_Final_of_MPC_Bandwidth_Result_UnbalancedNew/Subsystem1/ModulatorTimes/ConverterVoltage/DQConvSector5 ==
  MPCC_f32ElectricalAngle_K_1 : Inport
  MPCC_f32AlphaConvVoltage5 : Inport  Port=2
  MPCC_f32BetaConvVoltage5 : Inport  Port=3
  MPCC_f32AlphaConvVoltage6 : Inport  Port=4
  MPCC_f32BetaConvVoltage6 : Inport  Port=5
  MPCC_f32Duty_Sector5 : Inport  Port=6
  Add : Sum  Commented=on
  Add1 : Sum  Commented=on  Inputs=-+
  Add2 : Sum
  Add3 : Sum
  Demux : Demux
  From1 : From  Commented=on  GotoTag=MPCC_f32AlphaConvSector5
  From2 : From  Commented=on  GotoTag=MPCC_f32BetaConvSector5
  From{3,6..8} (4 alike) : From  Commented=on  GotoTag=MPCC_f32ElectricalAngle_K_1
  From4 : From  Commented=on  GotoTag=MPCC_f32AlphaConvSector5
  From5 : From  Commented=on  GotoTag=MPCC_f32BetaConvSector5
  Product{,1..3} (4 alike) : Product  Commented=on
  Product{4..7} (4 alike) : Product
  Sin : Trigonometry  Commented=on  Operator=cos
  Sin1 : Trigonometry  Commented=on
  Sin2 : Trigonometry  Commented=on
  Sin3 : Trigonometry  Commented=on  Operator=cos
  MPCC_f32DConvSector5 : Outport
  MPCC_f32QConvSector5 : Outport  Port=2
  wires:
  Sin2/1 -> Product2/1
  From5/1 -> Product3/2
  Sin1/1 -> Product1/1
  Sin3/1 -> Product3/1
  Product/1 -> Add/1
  From4/1 -> Product2/2
  From8/1 -> Sin2/1
  From2/1 -> Product1/2
  Product2/1 -> Add1/1
  Product3/1 -> Add1/2
  From6/1 -> Sin3/1
  MPCC_f32ElectricalAngle_K_1/1 -> [MPCC_f32ElectricalAngle_K_1]
  From7/1 -> Sin/1
  From1/1 -> Product/2
  Product1/1 -> Add/2
  Sin/1 -> Product/1
  From3/1 -> Sin1/1
  MPCC_f32AlphaConvVoltage5/1 -> [MPCC_f32AlphaConvVoltage5]
  MPCC_f32BetaConvVoltage5/1 -> [MPCC_f32BetaConvVoltage5]
  MPCC_f32AlphaConvVoltage6/1 -> [MPCC_f32AlphaConvVoltage6]
  MPCC_f32BetaConvVoltage6/1 -> [MPCC_f32BetaConvVoltage6]
  [MPCC_f32DutyA_Sector5] -> Product4/1
  [MPCC_f32DutyB_Sector5] -> Product5/1
  [MPCC_f32AlphaConvVoltage5] -> Product4/2
  Product4/1 -> Add2/1
  [MPCC_f32AlphaConvVoltage6] -> Product5/2
  Product5/1 -> Add2/2
  [MPCC_f32DutyB_Sector5] -> Product7/1
  [MPCC_f32DutyA_Sector5] -> Product6/1
  [MPCC_f32BetaConvVoltage6] -> Product7/2
  Product6/1 -> Add3/1
  Product7/1 -> Add3/2
  [MPCC_f32BetaConvVoltage5] -> Product6/2
  MPCC_f32Duty_Sector5/1 -> Demux/1
  Demux/1 -> [MPCC_f32DutyA_Sector5]
  Demux/2 -> [MPCC_f32DutyB_Sector5]
  Add3/1 -> MPCC_f32QConvSector5/1, [MPCC_f32BetaConvSector5]
  Add2/1 -> MPCC_f32DConvSector5/1, [MPCC_f32AlphaConvSector5]

== system AB_Final_of_MPC_Bandwidth_Result_UnbalancedNew/Subsystem1/ModulatorTimes/ConverterVoltage/DQConvSector6 ==
  MPCC_f32ElectricalAngle_K_1 : Inport
  MPCC_f32AlphaConvVoltage6 : Inport  Port=2
  MPCC_f32BetaConvVoltage6 : Inport  Port=3
  MPCC_f32AlphaConvVoltage1 : Inport  Port=4
  MPCC_f32BetaConvVoltage1 : Inport  Port=5
  MPCC_f32Duty_Sector6 : Inport  Port=6
  Add : Sum  Commented=on
  Add1 : Sum  Commented=on  Inputs=-+
  Add2 : Sum
  Add3 : Sum
  Demux : Demux
  From1 : From  Commented=on  GotoTag=MPCC_f32AlphaConvSector6
  From2 : From  Commented=on  GotoTag=MPCC_f32BetaConvSector6
  From{3,6..8} (4 alike) : From  Commented=on  GotoTag=MPCC_f32ElectricalAngle_K_1
  From4 : From  Commented=on  GotoTag=MPCC_f32AlphaConvSector6
  From5 : From  Commented=on  GotoTag=MPCC_f32BetaConvSector6
  Product{,1..3} (4 alike) : Product  Commented=on
  Product{4..7} (4 alike) : Product
  Sin : Trigonometry  Commented=on  Operator=cos
  Sin1 : Trigonometry  Commented=on
  Sin2 : Trigonometry  Commented=on
  Sin3 : Trigonometry  Commented=on  Operator=cos
  MPCC_f32DConvSector6 : Outport
  MPCC_f32QConvSector6 : Outport  Port=2
  wires:
  Sin2/1 -> Product2/1
  From5/1 -> Product3/2
  Sin1/1 -> Product1/1
  Sin3/1 -> Product3/1
  Product/1 -> Add/1
  From4/1 -> Product2/2
  From8/1 -> Sin2/1
  From2/1 -> Product1/2
  Product2/1 -> Add1/1
  Product3/1 -> Add1/2
  From6/1 -> Sin3/1
  MPCC_f32ElectricalAngle_K_1/1 -> [MPCC_f32ElectricalAngle_K_1]
  From7/1 -> Sin/1
  From1/1 -> Product/2
  Product1/1 -> Add/2
  Sin/1 -> Product/1
  From3/1 -> Sin1/1
  MPCC_f32AlphaConvVoltage6/1 -> [MPCC_f32AlphaConvVoltage6]
  MPCC_f32BetaConvVoltage6/1 -> [MPCC_f32BetaConvVoltage6]
  MPCC_f32AlphaConvVoltage1/1 -> [MPCC_f32AlphaConvVoltage1]
  MPCC_f32BetaConvVoltage1/1 -> [MPCC_f32BetaConvVoltage1]
  [MPCC_f32DutyA_Sector6] -> Product4/1
  [MPCC_f32DutyB_Sector6] -> Product5/1
  [MPCC_f32AlphaConvVoltage6] -> Product4/2
  Product4/1 -> Add2/1
  [MPCC_f32AlphaConvVoltage1] -> Product5/2
  Product5/1 -> Add2/2
  [MPCC_f32DutyB_Sector6] -> Product7/1
  [MPCC_f32DutyA_Sector6] -> Product6/1
  [MPCC_f32BetaConvVoltage1] -> Product7/2
  Product6/1 -> Add3/1
  Product7/1 -> Add3/2
  [MPCC_f32BetaConvVoltage6] -> Product6/2
  MPCC_f32Duty_Sector6/1 -> Demux/1
  Demux/1 -> [MPCC_f32DutyA_Sector6]
  Demux/2 -> [MPCC_f32DutyB_Sector6]
  Add2/1 -> MPCC_f32DConvSector6/1, [MPCC_f32AlphaConvSector6]
  Add3/1 -> MPCC_f32QConvSector6/1, [MPCC_f32BetaConvSector6]

== system AB_Final_of_MPC_Bandwidth_Result_UnbalancedNew/Subsystem1/PSCE/SOGI 1st4/Integrator ==
  In : Inport
  Delay1 : Delay  DelayLength=1
  Delay2 : Delay  DelayLength=1
  Delay3 : Delay  DelayLength=1
  Gain : Gain  Gain=100e-6/12
  Gain1 : Gain  Gain=23
  Gain2 : Gain  Gain=16
  Gain3 : Gain  Gain=5
  Sum : Sum  Inputs=|+-
  Sum1 : Sum  Inputs=|++
  Sum2 : Sum  Inputs=|++
  Out : Outport
  wires:
  Delay2/1 -> Gain2/1, Delay3/1
  Delay1/1 -> Sum2/2, Gain1/1, Delay2/1
  Delay3/1 -> Gain3/1
  Gain2/1 -> Sum/2
  Gain1/1 -> Sum/1
  Gain3/1 -> Sum1/2
  Sum/1 -> Sum1/1
  Gain/1 -> Sum2/1
  Sum2/1 -> Delay1/1
  In/1 -> Gain/1
  Sum1/1 -> Out/1

== system AB_Final_of_MPC_Bandwidth_Result_UnbalancedNew/Subsystem1/PSCE/SOGI 1st4/Integrator1 ==
  In : Inport
  Delay1 : Delay  DelayLength=1
  Delay2 : Delay  DelayLength=1
  Delay3 : Delay  DelayLength=1
  Gain : Gain  Gain=100e-6/12
  Gain1 : Gain  Gain=23
  Gain2 : Gain  Gain=16
  Gain3 : Gain  Gain=5
  Sum : Sum  Inputs=|+-
  Sum1 : Sum  Inputs=|++
  Sum2 : Sum  Inputs=|++
  Out : Outport
  wires:
  Delay2/1 -> Gain2/1, Delay3/1
  Delay1/1 -> Sum2/2, Gain1/1, Delay2/1
  Delay3/1 -> Gain3/1
  Gain2/1 -> Sum/2
  Gain1/1 -> Sum/1
  Gain3/1 -> Sum1/2
  Sum/1 -> Sum1/1
  Gain/1 -> Sum2/1
  Sum2/1 -> Delay1/1
  In/1 -> Gain/1
  Sum1/1 -> Out/1

== system AB_Final_of_MPC_Bandwidth_Result_UnbalancedNew/Subsystem1/PSCE/SOGI 1st4/Integrator2 ==
  In : Inport
  Delay1 : Delay  DelayLength=1
  Delay2 : Delay  DelayLength=1
  Delay3 : Delay  DelayLength=1
  Gain : Gain  Gain=100e-6/12
  Gain1 : Gain  Gain=23
  Gain2 : Gain  Gain=16
  Gain3 : Gain  Gain=5
  Sum : Sum  Inputs=|+-
  Sum1 : Sum  Inputs=|++
  Sum2 : Sum  Inputs=|++
  Out : Outport
  wires:
  In/1 -> Gain/1
  Delay2/1 -> Gain2/1, Delay3/1
  Delay1/1 -> Sum2/2, Gain1/1, Delay2/1
  Delay3/1 -> Gain3/1
  Gain2/1 -> Sum/2
  Gain1/1 -> Sum/1
  Gain3/1 -> Sum1/2
  Sum/1 -> Sum1/1
  Sum1/1 -> Out/1
  Gain/1 -> Sum2/1
  Sum2/1 -> Delay1/1

== system AB_Final_of_MPC_Bandwidth_Result_UnbalancedNew/Subsystem1/PSCE/SOGI 1st5/Integrator ==
  In : Inport
  Delay1 : Delay  DelayLength=1
  Delay2 : Delay  DelayLength=1
  Delay3 : Delay  DelayLength=1
  Gain : Gain  Gain=100e-6/12
  Gain1 : Gain  Gain=23
  Gain2 : Gain  Gain=16
  Gain3 : Gain  Gain=5
  Sum : Sum  Inputs=|+-
  Sum1 : Sum  Inputs=|++
  Sum2 : Sum  Inputs=|++
  Out : Outport
  wires:
  Delay2/1 -> Gain2/1, Delay3/1
  Delay1/1 -> Sum2/2, Gain1/1, Delay2/1
  Delay3/1 -> Gain3/1
  Gain2/1 -> Sum/2
  Gain1/1 -> Sum/1
  Gain3/1 -> Sum1/2
  Sum/1 -> Sum1/1
  Gain/1 -> Sum2/1
  Sum2/1 -> Delay1/1
  In/1 -> Gain/1
  Sum1/1 -> Out/1

== system AB_Final_of_MPC_Bandwidth_Result_UnbalancedNew/Subsystem1/PSCE/SOGI 1st5/Integrator1 ==
  In : Inport
  Delay1 : Delay  DelayLength=1
  Delay2 : Delay  DelayLength=1
  Delay3 : Delay  DelayLength=1
  Gain : Gain  Gain=100e-6/12
  Gain1 : Gain  Gain=23
  Gain2 : Gain  Gain=16
  Gain3 : Gain  Gain=5
  Sum : Sum  Inputs=|+-
  Sum1 : Sum  Inputs=|++
  Sum2 : Sum  Inputs=|++
  Out : Outport
  wires:
  Delay2/1 -> Gain2/1, Delay3/1
  Delay1/1 -> Sum2/2, Gain1/1, Delay2/1
  Delay3/1 -> Gain3/1
  Gain2/1 -> Sum/2
  Gain1/1 -> Sum/1
  Gain3/1 -> Sum1/2
  Sum/1 -> Sum1/1
  Gain/1 -> Sum2/1
  Sum2/1 -> Delay1/1
  In/1 -> Gain/1
  Sum1/1 -> Out/1

== system AB_Final_of_MPC_Bandwidth_Result_UnbalancedNew/Subsystem1/PSCE/SOGI 1st5/Integrator2 ==
  In : Inport
  Delay1 : Delay  DelayLength=1
  Delay2 : Delay  DelayLength=1
  Delay3 : Delay  DelayLength=1
  Gain : Gain  Gain=100e-6/12
  Gain1 : Gain  Gain=23
  Gain2 : Gain  Gain=16
  Gain3 : Gain  Gain=5
  Sum : Sum  Inputs=|+-
  Sum1 : Sum  Inputs=|++
  Sum2 : Sum  Inputs=|++
  Out : Outport
  wires:
  In/1 -> Gain/1
  Delay2/1 -> Gain2/1, Delay3/1
  Delay1/1 -> Sum2/2, Gain1/1, Delay2/1
  Delay3/1 -> Gain3/1
  Gain2/1 -> Sum/2
  Gain1/1 -> Sum/1
  Gain3/1 -> Sum1/2
  Sum/1 -> Sum1/1
  Sum1/1 -> Out/1
  Gain/1 -> Sum2/1
  Sum2/1 -> Delay1/1

== system AB_Final_of_MPC_Bandwidth_Result_UnbalancedNew/Subsystem1/PSCE1/SOGI 1st4/Integrator ==
  In : Inport
  Delay1 : Delay  DelayLength=1
  Delay2 : Delay  DelayLength=1
  Delay3 : Delay  DelayLength=1
  Gain : Gain  Gain=100e-6/12
  Gain1 : Gain  Gain=23
  Gain2 : Gain  Gain=16
  Gain3 : Gain  Gain=5
  Sum : Sum  Inputs=|+-
  Sum1 : Sum  Inputs=|++
  Sum2 : Sum  Inputs=|++
  Out : Outport
  wires:
  Delay2/1 -> Gain2/1, Delay3/1
  Delay1/1 -> Sum2/2, Gain1/1, Delay2/1
  Delay3/1 -> Gain3/1
  Gain2/1 -> Sum/2
  Gain1/1 -> Sum/1
  Gain3/1 -> Sum1/2
  Sum/1 -> Sum1/1
  Gain/1 -> Sum2/1
  Sum2/1 -> Delay1/1
  In/1 -> Gain/1
  Sum1/1 -> Out/1

== system AB_Final_of_MPC_Bandwidth_Result_UnbalancedNew/Subsystem1/PSCE1/SOGI 1st4/Integrator1 ==
  In : Inport
  Delay1 : Delay  DelayLength=1
  Delay2 : Delay  DelayLength=1
  Delay3 : Delay  DelayLength=1
  Gain : Gain  Gain=100e-6/12
  Gain1 : Gain  Gain=23
  Gain2 : Gain  Gain=16
  Gain3 : Gain  Gain=5
  Sum : Sum  Inputs=|+-
  Sum1 : Sum  Inputs=|++
  Sum2 : Sum  Inputs=|++
  Out : Outport
  wires:
  Delay2/1 -> Gain2/1, Delay3/1
  Delay1/1 -> Sum2/2, Gain1/1, Delay2/1
  Delay3/1 -> Gain3/1
  Gain2/1 -> Sum/2
  Gain1/1 -> Sum/1
  Gain3/1 -> Sum1/2
  Sum/1 -> Sum1/1
  Gain/1 -> Sum2/1
  Sum2/1 -> Delay1/1
  In/1 -> Gain/1
  Sum1/1 -> Out/1

== system AB_Final_of_MPC_Bandwidth_Result_UnbalancedNew/Subsystem1/PSCE1/SOGI 1st4/Integrator2 ==
  In : Inport
  Delay1 : Delay  DelayLength=1
  Delay2 : Delay  DelayLength=1
  Delay3 : Delay  DelayLength=1
  Gain : Gain  Gain=100e-6/12
  Gain1 : Gain  Gain=23
  Gain2 : Gain  Gain=16
  Gain3 : Gain  Gain=5
  Sum : Sum  Inputs=|+-
  Sum1 : Sum  Inputs=|++
  Sum2 : Sum  Inputs=|++
  Out : Outport
  wires:
  In/1 -> Gain/1
  Delay2/1 -> Gain2/1, Delay3/1
  Delay1/1 -> Sum2/2, Gain1/1, Delay2/1
  Delay3/1 -> Gain3/1
  Gain2/1 -> Sum/2
  Gain1/1 -> Sum/1
  Gain3/1 -> Sum1/2
  Sum/1 -> Sum1/1
  Sum1/1 -> Out/1
  Gain/1 -> Sum2/1
  Sum2/1 -> Delay1/1

== system AB_Final_of_MPC_Bandwidth_Result_UnbalancedNew/Subsystem1/PSCE1/SOGI 1st5/Integrator ==
  In : Inport
  Delay1 : Delay  DelayLength=1
  Delay2 : Delay  DelayLength=1
  Delay3 : Delay  DelayLength=1
  Gain : Gain  Gain=100e-6/12
  Gain1 : Gain  Gain=23
  Gain2 : Gain  Gain=16
  Gain3 : Gain  Gain=5
  Sum : Sum  Inputs=|+-
  Sum1 : Sum  Inputs=|++
  Sum2 : Sum  Inputs=|++
  Out : Outport
  wires:
  Delay2/1 -> Gain2/1, Delay3/1
  Delay1/1 -> Sum2/2, Gain1/1, Delay2/1
  Delay3/1 -> Gain3/1
  Gain2/1 -> Sum/2
  Gain1/1 -> Sum/1
  Gain3/1 -> Sum1/2
  Sum/1 -> Sum1/1
  Gain/1 -> Sum2/1
  Sum2/1 -> Delay1/1
  In/1 -> Gain/1
  Sum1/1 -> Out/1

== system AB_Final_of_MPC_Bandwidth_Result_UnbalancedNew/Subsystem1/PSCE1/SOGI 1st5/Integrator1 ==
  In : Inport
  Delay1 : Delay  DelayLength=1
  Delay2 : Delay  DelayLength=1
  Delay3 : Delay  DelayLength=1
  Gain : Gain  Gain=100e-6/12
  Gain1 : Gain  Gain=23
  Gain2 : Gain  Gain=16
  Gain3 : Gain  Gain=5
  Sum : Sum  Inputs=|+-
  Sum1 : Sum  Inputs=|++
  Sum2 : Sum  Inputs=|++
  Out : Outport
  wires:
  Delay2/1 -> Gain2/1, Delay3/1
  Delay1/1 -> Sum2/2, Gain1/1, Delay2/1
  Delay3/1 -> Gain3/1
  Gain2/1 -> Sum/2
  Gain1/1 -> Sum/1
  Gain3/1 -> Sum1/2
  Sum/1 -> Sum1/1
  Gain/1 -> Sum2/1
  Sum2/1 -> Delay1/1
  In/1 -> Gain/1
  Sum1/1 -> Out/1

== system AB_Final_of_MPC_Bandwidth_Result_UnbalancedNew/Subsystem1/PSCE1/SOGI 1st5/Integrator2 ==
  In : Inport
  Delay1 : Delay  DelayLength=1
  Delay2 : Delay  DelayLength=1
  Delay3 : Delay  DelayLength=1
  Gain : Gain  Gain=100e-6/12
  Gain1 : Gain  Gain=23
  Gain2 : Gain  Gain=16
  Gain3 : Gain  Gain=5
  Sum : Sum  Inputs=|+-
  Sum1 : Sum  Inputs=|++
  Sum2 : Sum  Inputs=|++
  Out : Outport
  wires:
  In/1 -> Gain/1
  Delay2/1 -> Gain2/1, Delay3/1
  Delay1/1 -> Sum2/2, Gain1/1, Delay2/1
  Delay3/1 -> Gain3/1
  Gain2/1 -> Sum/2
  Gain1/1 -> Sum/1
  Gain3/1 -> Sum1/2
  Sum/1 -> Sum1/1
  Sum1/1 -> Out/1
  Gain/1 -> Sum2/1
  Sum2/1 -> Delay1/1

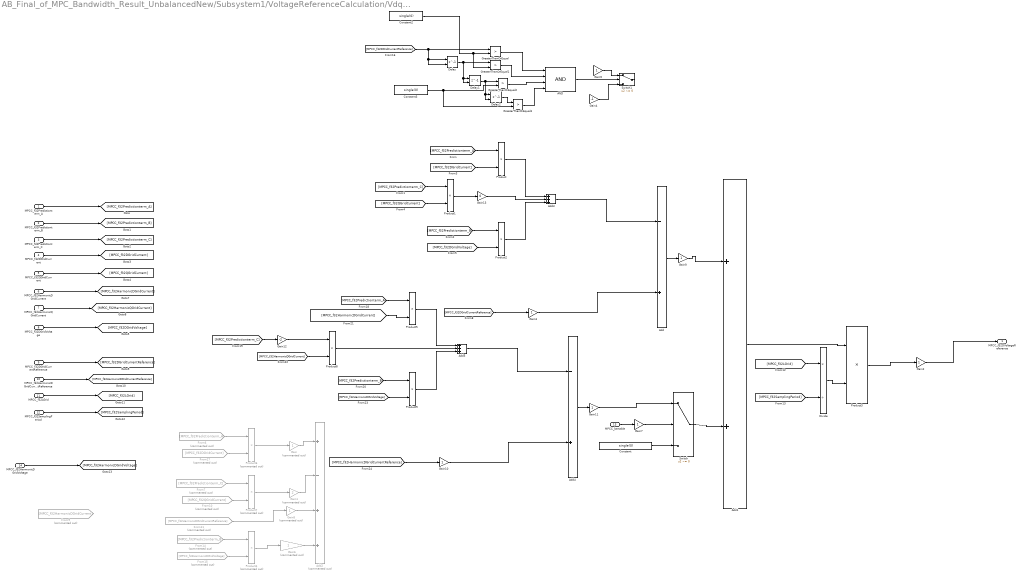
== system AB_Final_of_MPC_Bandwidth_Result_UnbalancedNew/Subsystem1/VoltageReferenceCalculation/VdqVoltageReferenceCalculation/VdVoltageReferenceCalculation ==
  MPCC_f32Predictionterm_A : Inport
  MPCC_f32Predictionterm_B : Inport  Port=2
  MPCC_f32Predictionterm_C : Inport  Port=3
  MPCC_f32DGridCurrent : Inport  Port=4
  MPCC_f32QGridCurrent : Inport  Port=5
  MPCC_f32HarmonicDGridCurrent : Inport  Port=6
  MPCC_f32HarmonicQGridCurrent : Inport  Port=7
  MPCC_f32DGridVoltage : Inport  Port=8
  MPCC_f32DGridCurrentReference : Inport  Port=9
  MPCC_f32HarmonicDGridCurrentReference : Inport  Port=10
  MPCC_f32LGrid : Inport  Port=11
  MPCC_f32SamplingPeriod : Inport  Port=12
  MPCC_benable : Inport  Port=13
  MPCC_f32HarmonicDGridVoltage : Inport  Port=14
  AND : Logic  Inputs=4  AllPortsSameDT=off  OutDataTypeStr=boolean
  Add : Sum  Inputs=-+
  Add1 : Sum
  Add2 : Sum  Commented=on  Inputs=+-++
  Add3 : Sum  Inputs=+++
  Add4 : Sum  Inputs=-+
  Add5 : Sum  Inputs=+++
  Constant : Constant  Value=single(0)
  Constant2 : Constant  Value=single(0)
  Constant3 : Constant  Value=single(0)
  Delay : Delay  DelayLength=1  InitialConditionSource=Input port
      settings: InputPortMap=u0,p4
  Delay1 : Delay  DelayLength=1  InitialConditionSource=Input port
      settings: InputPortMap=u0,p4
  Delay2 : Delay  DelayLength=1  InitialConditionSource=Input port
      settings: InputPortMap=u0,p4
  Divide : Product  Inputs=*/  RndMeth=Zero  SaturateOnIntegerOverflow=on
  From10 : From  Commented=on  GotoTag=MPCC_f32QGridCurrent
  From11 : From  Commented=on  GotoTag=MPCC_f32HarmonicDGridCurrentReference
  From14 : From  Commented=on  GotoTag=MPCC_f32Predictionterm_B
  From15 : From  Commented=on  GotoTag=MPCC_f32HarmonicDGridVoltage
  From17 : From  Commented=on  GotoTag=MPCC_f32DGridCurrent
  From6 : From  Commented=on  GotoTag=MPCC_f32Predictionterm_A
  From7 : From  Commented=on  GotoTag=MPCC_f32Predictionterm_C
  From9 : From  Commented=on  GotoTag=MPCC_f32HarmonicDGridCurrent
  Gain : Gain  Commented=on
  Gain1 : Gain  Commented=on  Gain=2
  Gain{2..3,5,7,9..11} (7 alike) : Gain
  Gain12 : Gain  Gain=-2
  Gain13 : Gain  Gain=0
  Gain4 : Gain  Gain=-1
  Gain6 : Gain  Commented=on
  Gain8 : Gain  Commented=on
  GreaterThanOrEqual{,1..3} (4 alike) : RelationalOperator  Operator=>  OutDataTypeStr=boolean  RndMeth=Simplest  InputSameDT=off
  Product : Product
  Product{1..2,8..9} (4 alike) : Product  OutDataTypeStr=Inherit: Inherit via back propagation
  Product3 : Product
  Product4 : Product  Commented=on  OutDataTypeStr=Inherit: Inherit via back propagation
  Product5 : Product
  Product6 : Product  Commented=on
  Product7 : Product  Commented=on
  Switch : Switch  Criteria=u2 ~= 0  SaturateOnIntegerOverflow=off  InputSameDT=off
  Switch1 : Switch  Criteria=u2 ~= 0  SaturateOnIntegerOverflow=off  InputSameDT=off
  MPCC_f32DVoltageReference : Outport
  wires:
  MPCC_f32Predictionterm_A/1 -> [MPCC_f32Predictionterm_A]
  MPCC_f32Predictionterm_B/1 -> [MPCC_f32Predictionterm_B]
  MPCC_f32Predictionterm_C/1 -> [MPCC_f32Predictionterm_C]
  MPCC_f32DGridCurrent/1 -> [MPCC_f32DGridCurrent]
  MPCC_f32QGridCurrent/1 -> [MPCC_f32QGridCurrent]
  MPCC_f32HarmonicDGridCurrent/1 -> [MPCC_f32HarmonicDGridCurrent]
  MPCC_f32HarmonicQGridCurrent/1 -> [MPCC_f32HarmonicQGridCurrent]
  MPCC_f32DGridVoltage/1 -> [MPCC_f32DGridVoltage]
  Constant/1 -> Switch/3
  MPCC_benable/1 -> Gain7/1
  Switch/1 -> Add1/2
  Add/1 -> Gain9/1
  MPCC_f32DGridCurrentReference/1 -> [MPCC_f32DGridCurrentReference]
  MPCC_f32HarmonicDGridCurrentReference/1 -> [MPCC_f32HarmonicDGridCurrentReference]
  [MPCC_f32DGridCurrentReference] -> Gain3/1
  MPCC_f32LGrid/1 -> [MPCC_f32LGrid]
  MPCC_f32SamplingPeriod/1 -> [MPCC_f32SamplingPeriod]
  [MPCC_f32LGrid] -> Divide/1
  [MPCC_f32SamplingPeriod] -> Divide/2
  Divide/1 -> Product3/2
  Product3/1 -> Gain2/1
  Gain2/1 -> MPCC_f32DVoltageReference/1
  [MPCC_f32QGridCurrent] -> Product1/2
  [MPCC_f32Predictionterm_C] -> Product1/1
  [MPCC_f32DGridVoltage] -> Product2/2
  [MPCC_f32Predictionterm_B] -> Product2/1
  [MPCC_f32DGridCurrent] -> Product/2
  [MPCC_f32Predictionterm_A] -> Product/1
  Product/1 -> Add3/1
  Product1/1 -> Gain13/1
  Product2/1 -> Add3/3
  Gain3/1 -> Add/2
  Constant2/1 -> GreaterThanOrEqual1/2, GreaterThanOrEqual/2
  Delay/1 -> GreaterThanOrEqual1/1, Delay1/2, Delay1/1
  Constant3/1 -> GreaterThanOrEqual3/2, GreaterThanOrEqual2/2
  Delay1/1 -> Delay2/2, Delay2/1, GreaterThanOrEqual2/1
  [MPCC_f32DGridCurrentReference] -> GreaterThanOrEqual/1, Delay/2, Delay/1
  GreaterThanOrEqual3/1 -> AND/4
  GreaterThanOrEqual/1 -> AND/1
  Delay2/1 -> GreaterThanOrEqual3/1
  GreaterThanOrEqual1/1 -> AND/2
  GreaterThanOrEqual2/1 -> AND/3
  AND/1 -> Switch1/2
  Gain4/1 -> Switch1/3
  Gain5/1 -> Switch1/1
  Add1/1 -> Product3/1
  Add3/1 -> Add/1
  MPCC_f32HarmonicDGridVoltage/1 -> [MPCC_f32HarmonicDGridVoltage]
  Gain7/1 -> Switch/2
  Gain9/1 -> Add1/1
  Gain8/1 -> Add2/3
  Gain/1 -> Add2/1
  Gain6/1 -> Add2/4
  From14/1 -> Product4/1
  From15/1 -> Product4/2
  From17/1 -> Product6/2
  From6/1 -> Product6/1
  Product6/1 -> Gain/1
  From11/1 -> Gain8/1
  Product7/1 -> Gain1/1
  Gain1/1 -> Add2/2
  From10/1 -> Product7/2
  Product4/1 -> Gain6/1
  From7/1 -> Product7/1
  Gain11/1 -> Switch/1
  Add5/1 -> Add4/1
  [MPCC_f32HarmonicDGridCurrentReference] -> Gain10/1
  Add4/1 -> Gain11/1
  Product5/1 -> Add5/1
  Gain10/1 -> Add4/2
  [MPCC_f32Predictionterm_C] -> Gain12/1
  [MPCC_f32HarmonicDGridCurrent] -> Product5/2
  [MPCC_f32Predictionterm_B] -> Product9/1
  [MPCC_f32HarmonicQGridCurrent] -> Product8/2
  Product8/1 -> Add5/2
  Product9/1 -> Add5/3
  [MPCC_f32Predictionterm_A] -> Product5/1
  [MPCC_f32HarmonicDGridVoltage] -> Product9/2
  Gain12/1 -> Product8/1
  Gain13/1 -> Add3/2
